simulink model "teste2a"  (R2014a)
settings: Solver=ode3  StartTime=0.0  StopTime=80  FixedStep=0.001  RelTol=1e-3
libraries: commchan3 x1
settings Model: Creator=andre  LastModifiedBy=andre

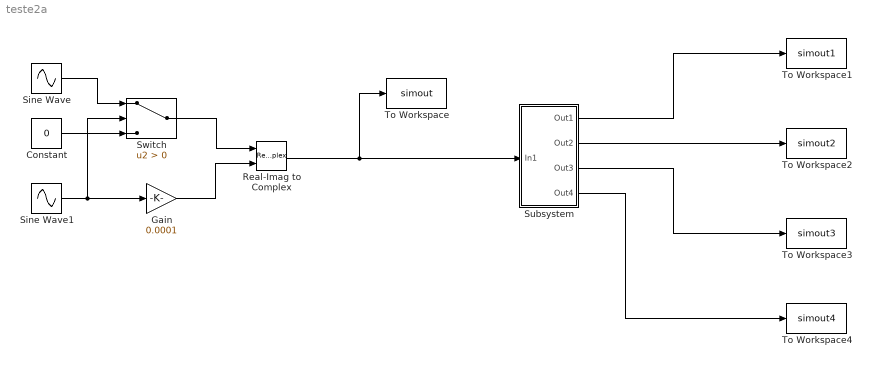
== system teste2a ==
  Constant : Constant  Value=0
  Gain : Gain  Gain=0.0001
  Real-Imag to Complex : RealImagToComplex
  Sine Wave : Sin  Frequency=10  Phase=0.15  SampleTime=0
  Sine Wave1 : Sin  SampleTime=0
  Subsystem : Subsystem
  Switch : Switch  Criteria=u2 > Threshold
  To Workspace : ToWorkspace  VariableName=simout  SampleTime=-1
  To Workspace1 : ToWorkspace  VariableName=simout1  SampleTime=-1
  To Workspace2 : ToWorkspace  VariableName=simout2  SampleTime=-1
  To Workspace3 : ToWorkspace  VariableName=simout3  SampleTime=-1
  To Workspace4 : ToWorkspace  VariableName=simout4  SaveFormat=Timeseries  SampleTime=-1
  wires:
  Subsystem/2(Out2) -> To Workspace2/1
  Subsystem/3(Out3) -> To Workspace3/1
  Real-Imag to Complex/1 -> To Workspace/1, Subsystem/1(In1)
  Subsystem/1(Out1) -> To Workspace1/1
  Gain/1 -> Real-Imag to Complex/2
  Sine Wave/1 -> Switch/1
  Switch/1 -> Real-Imag to Complex/1
  Sine Wave1/1 -> Switch/2, Gain/1
  Constant/1 -> Switch/3
  Subsystem/4(Out4) -> To Workspace4/1

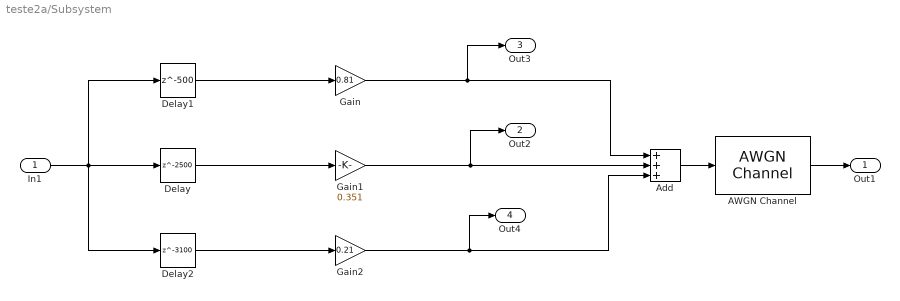
== system teste2a/Subsystem ==
  In1 : Inport
  AWGN Channel : commchan3/AWGN Channel  InputProcessing=Inherited (this choice will be removed - see release notes)  seed=67  noiseMode="Signal to noise ratio  (SNR)"  EbNodB=30  EsNodB=10  SNRdB=30  bitsPerSym=1  Ps=1  Tsym=1  variance=1
  Add : Sum  Inputs=+++
  Delay : Delay  DelayLength=2500
  Delay1 : Delay  DelayLength=500
  Delay2 : Delay  DelayLength=3100
  Gain : Gain  Gain=0.81
  Gain1 : Gain  Gain=0.351
  Gain2 : Gain  Gain=0.21
  Out1 : Outport
  Out2 : Outport  Port=2
  Out3 : Outport  Port=3
  Out4 : Outport  Port=4
  wires:
  AWGN Channel/1 -> Out1/1
  Add/1 -> AWGN Channel/1
  Gain1/1 -> Add/2, Out2/1
  Gain/1 -> Add/1, Out3/1
  Delay/1 -> Gain1/1
  Delay1/1 -> Gain/1
  Gain2/1 -> Out4/1, Add/3
  In1/1 -> Delay1/1, Delay2/1, Delay/1
  Delay2/1 -> Gain2/1
